simulink model "simPIDConv"  (R2020a)
settings: Solver=VariableStepAuto  StartTime=0.0  StopTime=80  RelTol=1e-3
values from neighbouring files (symbols this model uses):
  A = [0 1 0 0 ... (first row only)    [SystemModel.m]
  B = [0; 1/m1; 0; 0]    [SystemModel.m]
  C = [0 1 0 0]    [SystemModel.m]
  D = [0]    [SystemModel.m]
  Ts = 5e-03    (= 0.005)    [DataProcessingPIDConv.m]    (also in DataProcessingPIDConvFuzzy.m; DataProcessingPIDPSO.m; mainPSO.m = 0.1)
  x = data3.Swarm.Global.BestPosition    [DataProcessingPIDPSO.m]    (also in RandomParticlePosition.m = c*r1.*UB; pidcontroller.m = pidset.full_passenger)
libraries: simulink x2, sdolib x2
settings Model: Creator=TUF GAMING  LastModifiedBy=TUF GAMING

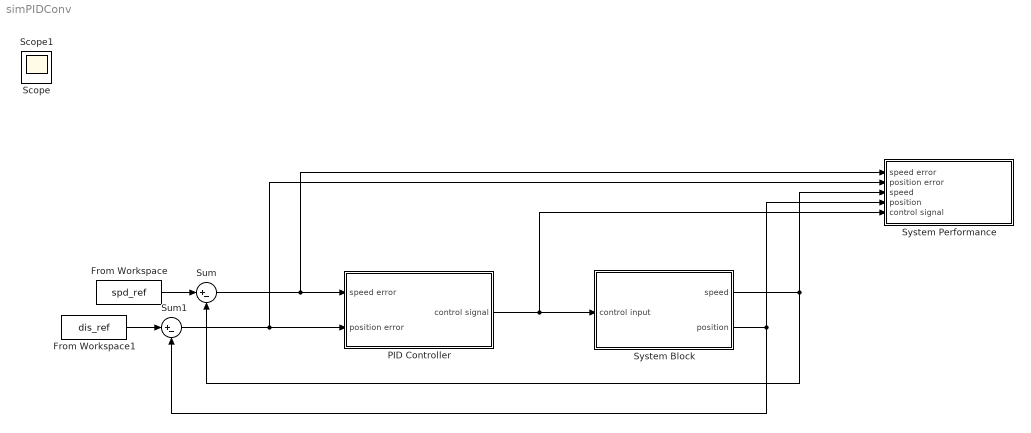
== system simPIDConv ==
  From Workspace : FromWorkspace  VariableName=spd_ref
  From Workspace1 : FromWorkspace  VariableName=dis_ref
  PID Controller : Subsystem
  Sum : Sum  Inputs=|+-
  Sum1 : Sum  Inputs=|+-
  System Block : Subsystem
  System Performance : Subsystem
  Scope : Scope
  Scope1 : Scope
  wires:
  From Workspace/1 -> Sum/1
  From Workspace1/1 -> Sum1/1
  Sum/1 -> PID Controller/1(speed error), System Performance/1(speed error)
  Sum1/1 -> PID Controller/2(position error), System Performance/2(position error)
  System Block/2(position) -> System Performance/4(position), Sum1/2
  System Block/1(speed) -> System Performance/3(speed), Sum/2
  PID Controller/1(control signal) -> System Block/1(control input), System Performance/5(control signal)

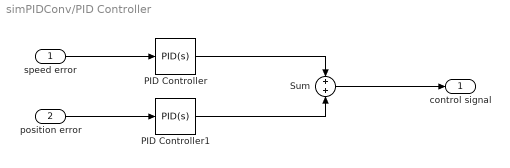
== system simPIDConv/PID Controller ==
  speed error : Inport
  position error : Inport  Port=2
  PID Controller : simulink/Continuous/PID Controller  Controller=PID  Form=Parallel  TimeDomain=Continuous-time  UseExternalTs=off  SampleTime=-1  IntegratorMethod=Forward Euler  FilterMethod=Forward Euler  ControllerParametersSource=internal  P=x(1)  I=x(2)  D=x(3)  UseFilter=on  N=100  TunerSelectOption=Transfer Function Based (PID Tuner App)  InitialConditionSource=internal  InitialConditionForIntegrator=0  InitialConditionForFilter=0  DifferentiatorICPrevScaledInput=0  ExternalReset=none  TrackingMode=off  Kt=1  LimitOutput=off  UpperSaturationLimit=inf  LowerSaturationLimit=-inf  LinearizeAsGain=on  AntiWindupMode=none  Kb=1  POutMin=[]  POutMax=[]  IOutMin=[]  IOutMax=[]  DOutMin=[]  DOutMax=[]  NOutMin=[]  NOutMax=[]  SumOutMin=[]  SumOutMax=[]  SaturationOutMin=[]  SaturationOutMax=[]  PParamMin=[]  PParamMax=[]  IParamMin=[]  IParamMax=[]  DParamMin=[]  DParamMax=[]  NParamMin=[]  NParamMax=[]  KbParamMin=[]  KbParamMax=[]  KtParamMin=[]  KtParamMax=[]  KbOutMin=[]  KbOutMax=[]  KtOutMin=[]  KtOutMax=[]  IntegratorOutMin=[]  IntegratorOutMax=[]  FilterOutMin=[]  FilterOutMax=[]  SumI1OutMin=[]  SumI1OutMax=[]  SumI2OutMin=[]  SumI2OutMax=[]  SumI3OutMin=[]  SumI3OutMax=[]  SumI4OutMin=[]  SumI4OutMax=[]  SumDOutMin=[]  SumDOutMax=[]  DifferentiatorOutMin=[]  DifferentiatorOutMax=[]  FilterDiffOutCoefMin=[]  FilterDiffOutCoefMax=[]  ReciprocalOutMin=[]  ReciprocalOutMax=[]  SumDenOutMin=[]  SumDenOutMax=[]  SumNumOutMin=[]  SumNumOutMax=[]  DivideOutMin=[]  DivideOutMax=[]  UdiffTsProdOutMin=[]  UdiffTsProdOutMax=[]  NTsProdOutMin=[]  NTsProdOutMax=[]  UintegralTsProdOutMin=[]  UintegralTsProdOutMax=[]  UngainTsProdOutMin=[]  UngainTsProdOutMax=[]  IntegratorContinuousStateAttributes=''  IntegratorStateMustResolveToSignalObject=off  IntegratorRTWStateStorageClass=Auto  FilterContinuousStateAttributes=''  FilterStateMustResolveToSignalObject=off  FilterRTWStateStorageClass=Auto  ParallelPVariant=InternalParameters  IdealPVariant=Disabled  IVariant=InternalParameters  DVariant=InternalParameters  IntegratorVariant=Continuous  SatVariant=Disabled  AWVariant=Passthrough  PCopyVariant=Disabled  TRVariant=Disabled  FdbkBlocksVariant=Forward  IdealPFdbkVariant=Disabled  SatFdbkVariant=Disabled  DerivativeFilterVariant=ContFilter  NVariant=InternalParameters  NCopyVariant=Disabled  FilterICVariant=InternalICsFilter  IntegratorICVariant=InternalICs  ExternalResetVariant=Disabled  TRSumVariant=Passthrough  SumFdbkVariant=Disabled  SumVariant=Sum_PID  TsampFilterVariant=InternalTs  TsampNgainVariant=Passthrough  TsampIntegralVariant=Passthrough
  PID Controller1 : simulink/Continuous/PID Controller  Controller=PID  Form=Parallel  TimeDomain=Continuous-time  UseExternalTs=off  SampleTime=-1  IntegratorMethod=Forward Euler  FilterMethod=Forward Euler  ControllerParametersSource=internal  P=x(4)  I=x(5)  D=x(6)  UseFilter=on  N=100  TunerSelectOption=Transfer Function Based (PID Tuner App)  InitialConditionSource=internal  InitialConditionForIntegrator=0  InitialConditionForFilter=0  DifferentiatorICPrevScaledInput=0  ExternalReset=none  TrackingMode=off  Kt=1  LimitOutput=off  UpperSaturationLimit=inf  LowerSaturationLimit=-inf  LinearizeAsGain=on  AntiWindupMode=none  Kb=1  POutMin=[]  POutMax=[]  IOutMin=[]  IOutMax=[]  DOutMin=[]  DOutMax=[]  NOutMin=[]  NOutMax=[]  SumOutMin=[]  SumOutMax=[]  SaturationOutMin=[]  SaturationOutMax=[]  PParamMin=[]  PParamMax=[]  IParamMin=[]  IParamMax=[]  DParamMin=[]  DParamMax=[]  NParamMin=[]  NParamMax=[]  KbParamMin=[]  KbParamMax=[]  KtParamMin=[]  KtParamMax=[]  KbOutMin=[]  KbOutMax=[]  KtOutMin=[]  KtOutMax=[]  IntegratorOutMin=[]  IntegratorOutMax=[]  FilterOutMin=[]  FilterOutMax=[]  SumI1OutMin=[]  SumI1OutMax=[]  SumI2OutMin=[]  SumI2OutMax=[]  SumI3OutMin=[]  SumI3OutMax=[]  SumI4OutMin=[]  SumI4OutMax=[]  SumDOutMin=[]  SumDOutMax=[]  DifferentiatorOutMin=[]  DifferentiatorOutMax=[]  FilterDiffOutCoefMin=[]  FilterDiffOutCoefMax=[]  ReciprocalOutMin=[]  ReciprocalOutMax=[]  SumDenOutMin=[]  SumDenOutMax=[]  SumNumOutMin=[]  SumNumOutMax=[]  DivideOutMin=[]  DivideOutMax=[]  UdiffTsProdOutMin=[]  UdiffTsProdOutMax=[]  NTsProdOutMin=[]  NTsProdOutMax=[]  UintegralTsProdOutMin=[]  UintegralTsProdOutMax=[]  UngainTsProdOutMin=[]  UngainTsProdOutMax=[]  IntegratorContinuousStateAttributes=''  IntegratorStateMustResolveToSignalObject=off  IntegratorRTWStateStorageClass=Auto  FilterContinuousStateAttributes=''  FilterStateMustResolveToSignalObject=off  FilterRTWStateStorageClass=Auto  ParallelPVariant=InternalParameters  IdealPVariant=Disabled  IVariant=InternalParameters  DVariant=InternalParameters  IntegratorVariant=Continuous  SatVariant=Disabled  AWVariant=Passthrough  PCopyVariant=Disabled  TRVariant=Disabled  FdbkBlocksVariant=Forward  IdealPFdbkVariant=Disabled  SatFdbkVariant=Disabled  DerivativeFilterVariant=ContFilter  NVariant=InternalParameters  NCopyVariant=Disabled  FilterICVariant=InternalICsFilter  IntegratorICVariant=InternalICs  ExternalResetVariant=Disabled  TRSumVariant=Passthrough  SumFdbkVariant=Disabled  SumVariant=Sum_PID  TsampFilterVariant=InternalTs  TsampNgainVariant=Passthrough  TsampIntegralVariant=Passthrough
  Sum : Sum
  control signal : Outport
  wires:
  speed error/1 -> PID Controller/1
  position error/1 -> PID Controller1/1
  PID Controller/1 -> Sum/1
  PID Controller1/1 -> Sum/2
  Sum/1 -> control signal/1

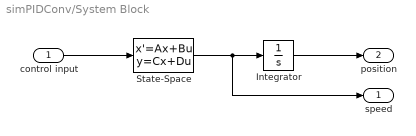
== system simPIDConv/System Block ==
  control input : Inport
  Integrator : Integrator
  State-Space : StateSpace  A=A  B=B  C=C  D=D  InitialCondition=0
  speed : Outport
  position : Outport  Port=2
  wires:
  State-Space/1 -> speed/1, Integrator/1
  Integrator/1 -> position/1
  control input/1 -> State-Space/1

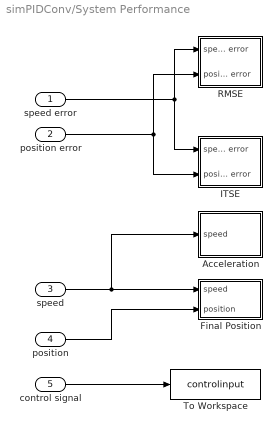
== system simPIDConv/System Performance ==
  speed error : Inport
  position error : Inport  Port=2
  speed : Inport  Port=3
  position : Inport  Port=4
  control signal : Inport  Port=5
  Acceleration : Subsystem
  Final Position : Subsystem
  ITSE : Subsystem
  RMSE : Subsystem
  To Workspace : ToWorkspace  VariableName=controlinput  SaveFormat=Timeseries  SampleTime=Ts
  wires:
  position error/1 -> RMSE/2(position error), ITSE/2(position error)
  speed error/1 -> RMSE/1(speed error), ITSE/1(speed error)
  position/1 -> Final Position/2(position)
  speed/1 -> Acceleration/1(speed), Final Position/1(speed)
  control signal/1 -> To Workspace/1

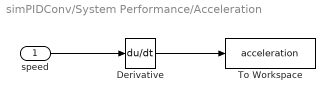
== system simPIDConv/System Performance/Acceleration ==
  speed : Inport
  Derivative : Derivative
  To Workspace : ToWorkspace  VariableName=acceleration  SaveFormat=Timeseries  SampleTime=Ts
  wires:
  Derivative/1 -> To Workspace/1
  speed/1 -> Derivative/1

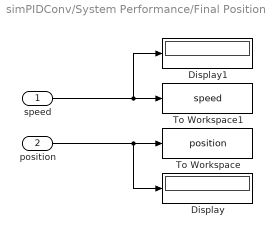
== system simPIDConv/System Performance/Final Position ==
  speed : Inport
  position : Inport  Port=2
  Display : Display
  Display1 : Display
  To Workspace : ToWorkspace  VariableName=position  SaveFormat=Timeseries  SampleTime=Ts
  To Workspace1 : ToWorkspace  VariableName=speed  SaveFormat=Timeseries  SampleTime=Ts
  wires:
  position/1 -> Display/1, To Workspace/1
  speed/1 -> Display1/1, To Workspace1/1

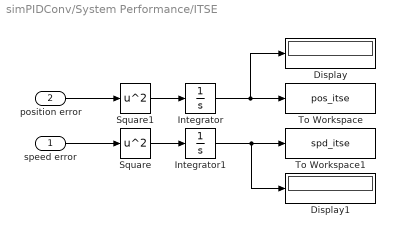
== system simPIDConv/System Performance/ITSE ==
  speed error : Inport
  position error : Inport  Port=2
  Display : Display
  Display1 : Display
  Integrator : Integrator
  Integrator1 : Integrator
  Square : Math  Operator=square  SaturateOnIntegerOverflow=on
  Square1 : Math  Operator=square  SaturateOnIntegerOverflow=on
  To Workspace : ToWorkspace  VariableName=pos_itse  SaveFormat=Timeseries  SampleTime=Ts
  To Workspace1 : ToWorkspace  VariableName=spd_itse  SaveFormat=Timeseries  SampleTime=Ts
  wires:
  Integrator1/1 -> To Workspace1/1, Display1/1
  Square1/1 -> Integrator/1
  Square/1 -> Integrator1/1
  Integrator/1 -> To Workspace/1, Display/1
  position error/1 -> Square1/1
  speed error/1 -> Square/1

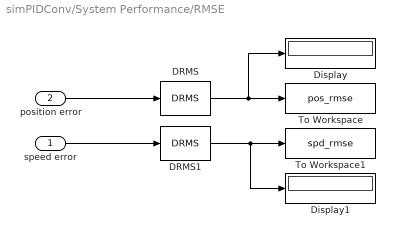
== system simPIDConv/System Performance/RMSE ==
  speed error : Inport
  position error : Inport  Port=2
  DRMS : sdolib/RMS Blocks/DRMS  Ts=Ts
      settings: SourceProductBaseCode=SO
  DRMS1 : sdolib/RMS Blocks/DRMS  Ts=Ts
      settings: SourceProductBaseCode=SO
  Display : Display
  Display1 : Display
  To Workspace : ToWorkspace  VariableName=pos_rmse  SaveFormat=Timeseries  SampleTime=Ts
  To Workspace1 : ToWorkspace  VariableName=spd_rmse  SaveFormat=Timeseries  SampleTime=Ts
  wires:
  DRMS1/1 -> To Workspace1/1, Display1/1
  DRMS/1 -> To Workspace/1, Display/1
  position error/1 -> DRMS/1
  speed error/1 -> DRMS1/1
